simulink model "mech_flyball"  (Simulink 6.0)
settings: Solver=ode15s  StartTime=0.0  StopTime=30  FixedStep=1e-2  RelTol=1e-3
PreLoadFcn:
  | flyball=mech_flyball_data;
InitFcn:
  | flyball=mech_flyball_data;
values from neighbouring files (symbols this model uses):
  m = 161    [mech_transmission_data.mat]
  N = 270    [mech_transmission_data.mat]
undefined symbols (not defined in the file or in its folder): mech_flyball_rod_inertia, mech_flyball_rod_mass, sigbuilder_block
libraries: mblibv1 x14, mech_flyball_lib x4
settings Model: Creator=nbrewton  LastModifiedBy=batserve  ExtModeAutoUpdateStatusClock=off
settings DataIOCC: MaxDataPoints=5000  SignalLoggingName=sigsOut
settings OptimizationCC: InlineInvariantSignals=off
settings DebuggingCC: CheckExecutionContextPreStartOutputMsg=on  CheckExecutionContextRuntimeOutputMsg=on  SolverPrmCheckMsg=none
settings HardwareCC: TargetHWDeviceType=MATLAB Host  ProdEqTarget=off
settings RTWCC: SystemTargetFile=rsim.tlc  TemplateMakefile=rsim_default_tmf  ProcessScript=rsim_make_rtw_hook
settings RSimTargetCC: TargetFcnLib=ansi_tfl_tmw.mat  GenFloatMathFcnCalls=ANSI_C  IsPILTarget=off
settings SimMechanicsCC: WarnOnRedundantConstraints=off  VisOnUpdateDiagram=on  VisDuringSimulation=on  VisConfigFile=mech_flyball_disp.mat

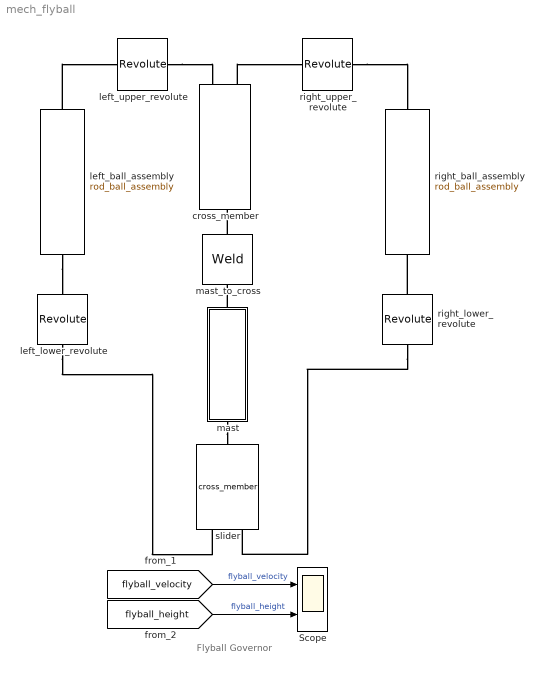
== system mech_flyball ==
  note: Flyball Governor
  Scope : Scope  NumInputPorts=2
      settings: YMin=0~-2.5  YMax=50~20
  cross_member : mech_flyball_lib/cross_member  Orientation=down  rod_length=flyball.cross_member.length  rod_radius=flyball.cross_member.radius  density=flyball.brass
  left_ball_assembly : mech_flyball_lib/rod_ball_assembly  Orientation=up  ball_radius=flyball.ball.radius  rod_radius=flyball.ball_rod.radius  rod_length=flyball.ball_rod.length  hookup_length=flyball.ball_rod.connection  density=flyball.brass  rotation=pi/4
  left_lower_revolute : mblibv1/Joints/Revolute  Orientation=up  PhysicalDomain=mechanical  SubClassName=Unknown  LeftPortType=blob  RightPortType=blob  LConnTagsString=__newl0  RConnTagsString=__newr0  NumSAPorts=0  CutJoint=off  MarkAsCut=off  Primitives=revolute  PrimitiveProps=R1$WORLD$[0 1 0]$revolute  DialogClass=JointBlock
  left_upper_revolute : mblibv1/Joints/Revolute  PhysicalDomain=mechanical  SubClassName=Unknown  LeftPortType=blob  RightPortType=blob  LConnTagsString=__newl0  RConnTagsString=__newr0  NumSAPorts=0  CutJoint=off  MarkAsCut=off  Primitives=revolute  PrimitiveProps=R1$WORLD$[0 1 0]$revolute  DialogClass=JointBlock
  mast : Subsystem  Orientation=up
  mast_to_cross : mblibv1/Joints/Weld  Orientation=up  PhysicalDomain=mechanical  SubClassName=Unknown  LeftPortType=blob  RightPortType=blob  LConnTagsString=__newl0  RConnTagsString=__newr0  NumSAPorts=0  CutJoint=off  MarkAsCut=off  Primitives=weld  PrimitiveProps=W$INERTIAL$[0 0 0]$weld  DialogClass=JointBlock
  right_ball_assembly : mech_flyball_lib/rod_ball_assembly  Orientation=up  ball_radius=flyball.ball.radius  rod_radius=flyball.ball_rod.radius  rod_length=flyball.ball_rod.length  hookup_length=flyball.ball_rod.connection  density=flyball.brass  rotation=-pi/4
  right_lower_revolute : mblibv1/Joints/Revolute  Orientation=up  PhysicalDomain=mechanical  SubClassName=Unknown  LeftPortType=blob  RightPortType=blob  LConnTagsString=__newl0  RConnTagsString=__newr0  NumSAPorts=0  CutJoint=off  MarkAsCut=off  Primitives=revolute  PrimitiveProps=R1$WORLD$[0 1 0]$revolute  DialogClass=JointBlock
  right_upper_revolute : mblibv1/Joints/Revolute  PhysicalDomain=mechanical  SubClassName=Unknown  LeftPortType=blob  RightPortType=blob  LConnTagsString=__newl0  RConnTagsString=__newr0  NumSAPorts=0  CutJoint=off  MarkAsCut=off  Primitives=revolute  PrimitiveProps=R1$WORLD$[0 1 0]$revolute  DialogClass=JointBlock
  slider : mech_flyball_lib/cross_member  Orientation=up  rod_length=flyball.cross_member.length  rod_radius=flyball.cross_member.radius  density=flyball.brass
  wires:
  [flyball_velocity] -> Scope/1  "flyball_velocity"
  [flyball_height] -> Scope/2  "flyball_height"
  connections:
  left_ball_assembly/RConn1 -- left_upper_revolute/LConn1
  left_upper_revolute/RConn1 -- cross_member/LConn1
  cross_member/LConn2 -- right_upper_revolute/LConn1
  right_upper_revolute/RConn1 -- right_ball_assembly/RConn1
  mast/LConn1 -- slider/RConn1
  left_lower_revolute/LConn1 -- slider/LConn1
  right_lower_revolute/RConn1 -- right_ball_assembly/LConn1
  right_lower_revolute/LConn1 -- slider/LConn2
  mast/RConn1 -- mast_to_cross/LConn1
  mast_to_cross/RConn1 -- cross_member/RConn1
  left_ball_assembly/LConn1 -- left_lower_revolute/RConn1

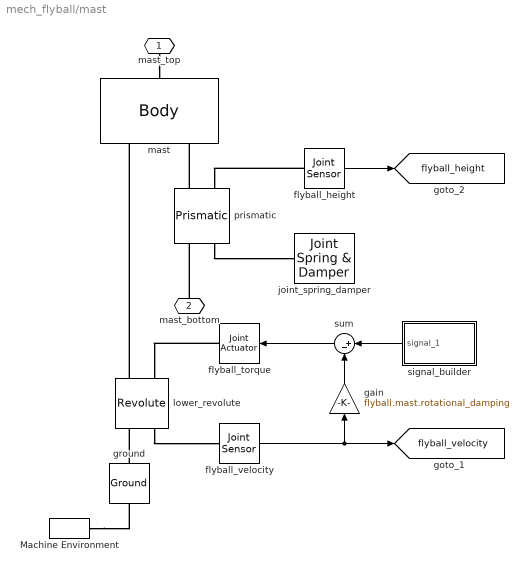
== system mech_flyball/mast ==
  Machine Environment : mblibv1/Bodies/Machine Environment  Tag=Factory ground  DialogController=MECH.DialogSource  Opaque=on  PortType=env  PhysicalDomain=Mechanical  DialogTemplateClass=MECH.MachineEnvironment  SyncWhenCopied=off  Gravity=[0 0 -9.81]  GravityUnits=m/s^2  GravityAsSignal=off  Dimensionality=3D Only  AnalysisType=Forward dynamics  LinearAssemblyTolerance=1e-3  LinearAssemblyToleranceUnits=m  AngularAssemblyTolerance=1e-3  AngularAssemblyToleranceUnits=rad  ConstraintSolverType=Stabilizing  ConstraintRelTolerance=1e-4  ConstraintAbsTolerance=1e-4  UseRobustSingularityHandling=off  StatePerturbationType=Fixed  PerturbationSize=1e-5  VisualizeMachine=on
  flyball_height : mblibv1/Sensors &  Actuators/Joint Sensor  Opaque=on  PhysicalDomain=Mechanical  PortType=blob  Muxed=on  Pose=off  Angle=on  AngleUnits=deg  ArcVelocity=off  ArcVelocityUnits=deg/s  ArcAcceleration=off  ArcAccelerationUnits=deg/s^2  CoordPosition=on  CoordPositionUnits=cm  Velocity=off  VelocityUnits=m/s  Acceleration=off  AccelerationUnits=m/s^2  Quaternion=on  QuaternionDT=off  QuaternionDDT=off  QuaternionUnits=deg  OutputVector=[ 1 ]  ActiveIO=on  Width=1  DialogClass=MechanicalSensorBlock  Primitive=P1  Force=off  ForceUnits=N  Torque=off  TorqueUnits=N-m  ReferenceFrame=Absolute (INERTIAL)  ReactionSensedSide=Base  ReactionReferenceFrame=Absolute (World)  ReactionForce=off  ReactionForceUnits=N  ReactionMoment=off  ReactionMomentUnits=N-m
  flyball_torque : mblibv1/Sensors &  Actuators/Joint Actuator  Orientation=left  Opaque=on  PhysicalDomain=Mechanical  PortType=blob  ActuationStyle=Force  AngleUnits=rad  ArcVelocityUnits=rad/s  ArcAccelerationUnits=rad/s^2  CoordPositionUnits=cm  VelocityUnits=cm/s  AccelerationUnits=cm/s^2  ForceUnits=N  TorqueUnits=N-m  ActiveIO=on  Width=1  DialogClass=MechanicalActuatorBlock  Primitive=R1  ReferenceFrame=Absolute (INERTIAL)
  flyball_velocity : mblibv1/Sensors &  Actuators/Joint Sensor  Opaque=on  PhysicalDomain=Mechanical  PortType=blob  Muxed=on  Pose=off  Angle=off  AngleUnits=deg  ArcVelocity=on  ArcVelocityUnits=rad/s  ArcAcceleration=off  ArcAccelerationUnits=deg/s^2  CoordPosition=on  CoordPositionUnits=m  Velocity=off  VelocityUnits=m/s  Acceleration=off  AccelerationUnits=m/s^2  Quaternion=on  QuaternionDT=off  QuaternionDDT=off  QuaternionUnits=deg  OutputVector=[ 1 ]  ActiveIO=on  Width=1  DialogClass=MechanicalSensorBlock  Primitive=R1  Force=off  ForceUnits=N  Torque=off  TorqueUnits=N-m  ReferenceFrame=Absolute (INERTIAL)  ReactionSensedSide=Base  ReactionReferenceFrame=Absolute (World)  ReactionForce=off  ReactionForceUnits=N  ReactionMoment=off  ReactionMomentUnits=N-m
  gain : Gain  Orientation=up  Gain=flyball.mast.rotational_damping  SaturateOnIntegerOverflow=on
  ground : mblibv1/Bodies/Ground  Orientation=up  Opaque=on  LeftPortType=env  RightPortType=workingframe  PhysicalDomain=Mechanical  DialogClass=GroundBlock  CoordPosition=[0 0 0]  CoordPositionUnits=m  StateVectorMgrId=-1  MachineId=[0 0]  ShowEnvPort=on
  joint_spring_damper : mblibv1/Force  Elements/Joint Spring & Damper  DialogClass=JointSpringDamper  JFEParameters=P1$true$flyball.mast.spring$flyball.mast.damping$0$cm$cm/s$N$rad$rad/s$N-m#P2$false$0$0$0$m$m/s$N$rad$rad/s$N-m#P3$false$0$0$0$m$m/s$N$rad$rad/s$N-m#R1$false$0$0$0$m$m/s$N$rad$rad/s$N-m#R2$false$0$0$0$m$m/s$N$rad$rad/s$N-m#R3$false$0$0$0$m$m/s$N$rad$rad/s$N-m#S$false$0$0$0$m$m/s$N$rad$rad/s$N-m
  lower_revolute : mblibv1/Joints/Revolute  Orientation=up  PhysicalDomain=mechanical  SubClassName=Unknown  LeftPortType=blob  RightPortType=blob  LConnTagsString=__newl0|SA1  RConnTagsString=__newr0|SA1  NumSAPorts=2  CutJoint=off  MarkAsCut=off  Primitives=revolute  PrimitiveProps=R1$WORLD$[0 0 1]$revolute  DialogClass=JointBlock
  mast : mblibv1/Bodies/Body  Orientation=up  PhysicalDomain=mechanical  SubClassName=Unknown  LeftPortType=workingframe  RightPortType=workingframe  LConnTagsString=CS1|CS3  RConnTagsString=CS2  DialogClass=MechanicalBodyBlock  Mass=mech_flyball_rod_mass(flyball.mast.length, flyball.mast.radius, flyball.brass)  MassUnits=g  InertiaUnits=g*cm^2  Inertia=mech_flyball_rod_inertia(flyball.mast.length, flyball.mast.radius, flyball.brass, [0 0 1])  Shape=Cylinder  ShapeDims=[1 1]  ShapeUnits=m  ShapeUse=false  Density=1  DensityUnits=kg/m^3  DensityUse=false  CG=Left$CG$[0 0 flyball.mast.length]*0.5$CS1$CS1$cm$[0 0 0]$Euler X-Y-Z$deg$WORLD$false  WorkingFrames=Left$CS1$[0 0 0]$ADJOINING$ADJOINING$cm$[0 0 0]$Euler X-Y-Z$deg$WORLD$true#Right$CS2$[0 0 flyball.mast.length]$CS1$CS1$cm$[0 0 0]$Euler X-Y-Z$deg$WORLD$true#Left$CS3$-[0 0 flyball.mast.connection]$CS2$CS2$cm$[0 0 0]$Euler X-Y-Z$deg$WORLD$true
  prismatic : mblibv1/Joints/Prismatic  Orientation=down  PhysicalDomain=mechanical  SubClassName=Unknown  LeftPortType=blob  RightPortType=blob  LConnTagsString=__newl0|SA1  RConnTagsString=__newr0|SA1  NumSAPorts=2  CutJoint=off  MarkAsCut=off  Primitives=prismatic  PrimitiveProps=P1$WORLD$[0 0 1]$prismatic  DialogClass=JointBlock
  signal_builder : Subsystem  Tag=STV Subsys  Orientation=left  LoadFcn=sigbuilder_block('load');  StartFcn=sigbuilder_block('start');  StopFcn=sigbuilder_block('stop');  ClipboardFcn=sigbuilder_block('clipboard');  mask(Sigbuilder block){}
      mask help: Sigbuilder GUI
      mask init:
      | if ~strcmp(get_param(bdroot(gcb),'SimulationStatus'),'stopped') tuvar = sigbuilder_block('maskInit'); end
      settings: CopyFcn=sigbuilder_block('copy');  DeleteFcn=sigbuilder_block('delete');  ModelCloseFcn=sigbuilder_block('modelClose');  PreSaveFcn=sigbuilder_block('preSave');  NameChangeFcn=sigbuilder_block('namechange');  OpenFcn=sigbuilder_block('open',[126.4 317.6 520 400 ]);  CloseFcn=sigbuilder_block('close');
      mask Display: plot(0,0,100,100,[10,10,40,40,10],[80,20,20,80,80],[40,10],[50,50], [40,27,10],[65,72,56],[40,25,25,10],[28,28,43,43]);
  sum : Sum  Orientation=left  Inputs=|+-  SaturateOnIntegerOverflow=on
  mast_top : PMIOPort  Orientation=down  Port=1  Side=Right
  mast_bottom : PMIOPort  Orientation=up  Port=2  Side=Left
  tag scope: flyball_height=global, flyball_velocity=global
  wires:
  sum/1 -> flyball_torque/1
  signal_builder/1(signal_1) -> sum/1
  flyball_velocity/1 -> gain/1, [flyball_velocity]
  gain/1 -> sum/2
  flyball_height/1 -> [flyball_height]
  connections:
  ground/RConn1 -- lower_revolute/LConn1
  prismatic/LConn1 -- mast/LConn2
  lower_revolute/RConn1 -- mast/LConn1
  mast_top/RConn1 -- mast/RConn1
  mast_bottom/RConn1 -- prismatic/RConn1
  prismatic/RConn2 -- joint_spring_damper/LConn1
  flyball_torque/RConn1 -- lower_revolute/RConn2
  lower_revolute/LConn2 -- flyball_velocity/LConn1
  flyball_height/LConn1 -- prismatic/LConn2
  Machine Environment/RConn1 -- ground/LConn1

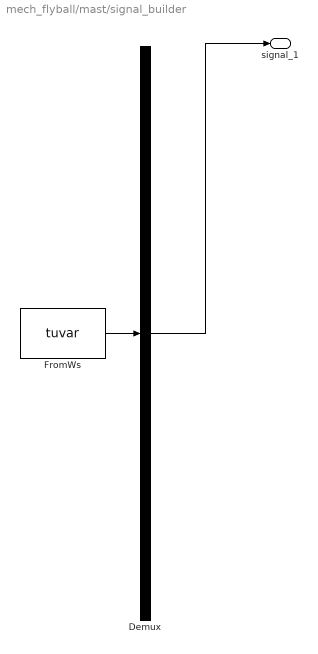
== system mech_flyball/mast/signal_builder ==
  Demux : Demux  Tag=STV Demux  Outputs=1
  FromWs : FromWorkspace  Tag=STV FromWs  VariableName=tuvar  SampleTime=0  SigBuilderData=DataTag1  VnvData=DataTag2
      SigBuilderData=|
      | channels.label = 'signal_1'
      | channels.allXData = {[0 5 5 5.05 5.05 20 20 20.05 20.05 30]}
      | channels.allYData = {[15 15 30 30 30 30 20 20 10 10]}
      | dataSet.timeRange = [0 30]
      | dataSet.name = 'Group 1'
  signal_1 : Outport  Tag=STV Outport
  wires:
  FromWs/1 -> Demux/1
  Demux/1 -> signal_1/1
